simulink model "Sim_PMSM"  (R2023a)
settings: Solver=ode45  StartTime=0  StopTime=Stop_Time  MaxStep=Ts  RelTol=1e-3  EnableMultiTasking=on
values from neighbouring files (symbols this model uses):
  Bm = .018    (= 0.018)    [A_PMSM.m]
  Jm = 0.01    [A_PMSM.m]
  Lamf = 0.254    [A_PMSM.m]
  Lamf_Hat = 1.0*Lamf    (= 0.254)    [A_PMSM.m]
  Lds = 3.6e-3    (= 0.0036)    [A_PMSM.m]
  Lds_Hat = 1.0*Lds    (= 0.0036)    [A_PMSM.m]
  Lqs = 4.3e-3    (= 0.0043)    [A_PMSM.m]
  Lqs_Hat = 1.0*Lqs    (= 0.0043)    [A_PMSM.m]
  p = 3    [A_PMSM.m]
  Rs = 0.15    [A_PMSM.m]
  Step_Time = [0.1 0.2 0.3 0.4]    [A_PMSM.m]
  Stop_Time = 0.5    [A_PMSM.m]
  Te_Rated = interp1(MTPA.Is(Ind_PosTe),MTPA.Te(Ind_PosTe),Is_Rated)    [A_PMSM.m]
  Te_Ref_Set = ones(1,5)*Te_Rated    [A_PMSM.m]
  Te_SlewRate = inf    [A_PMSM.m]
  Thetarm_Init = 0*pi*1/p    (= 0)    [A_PMSM.m]
  TL = zeros(1,5)    [A_PMSM.m]
  Ts = 1/fs    (= 5e-05)    [A_PMSM.m]
  Tsw = 1/fsw    (= 0.0001)    [A_PMSM.m]
  Vdc = 310    [A_PMSM.m]
  Wrm_Fin = 10000*2*pi/60    (= 1047.1975512)    [A_PMSM.m]
  Wrm_Init = Wrpm_Ref_Set(1)*2*pi/60    [A_PMSM.m]
  Wrpm_Ref_Set = Wrm_Init*ones(1,5)    [A_PMSM.m]
undefined symbols (not defined in the file or in its folder): CC, DiscIntNeverNeededParam, FW, Mode, MTPA, SC
libraries: simulink x6
settings Model: SimulationMode=accelerator  Creator=KYC  LastModifiedBy=INHA
settings SolverCC: AlgebraicLoopSolver=TrustRegion
settings DataIOCC: LimitDataPoints=on  SaveFormat=Array  ReturnWorkspaceOutputs=off
settings OptimizationCC: LifeSpan=inf
settings DebuggingCC: UnderspecifiedInitializationDetection=Classic  MergeDetectMultiDrivingBlocksExec=none  SolverPrmCheckMsg=warning  InheritedTsInSrcMsg=none  UnconnectedInputMsg=warning  UnconnectedOutputMsg=warning  UnconnectedLineMsg=warning  AllowSymbolicDim=off  StateNameClashWarn=warning  SFUnexpectedBacktrackingDiag=warning  SFNoUnconditionalDefaultTransitionDiag=warning  SFExecutionAtInitializationDiag=none  ArithmeticOperatorsInVariantConditions=warning
settings HardwareCC: ProdBitPerPointer=32  ProdBitPerSizeT=32  ProdBitPerPtrDiffT=32  ProdLargestAtomicFloat=None  ProdIntDivRoundTo=Undefined  ProdEndianess=Unspecified  ProdWordSize=32  ProdHWDeviceType=32-bit Generic
settings ModelReferenceCC: EnableRefExpFcnMdlSchedulingChecks=on  PropagateSignalLabelsOutOfModel=off
settings SFSimCC: SimUseLocalCustomCode=off  CustomCodeUndefinedFunction=UseInterfaceOnly
settings RTWCC: RTWUseLocalCustomCode=off
settings CodeAppCC: StateflowObjectComments=on
settings GRTTargetCC: TargetLangStandard=C89/C90 (ANSI)
settings ConfigComp: CovMetricSettings=dw  CovSaveCumulativeToWorkspaceVar=on  CovSaveSingleToWorkspaceVar=on  CovExternalEMLEnable=off  CovSFcnEnable=off
settings SimscapeCC: SimscapeNormalizeSystem=off

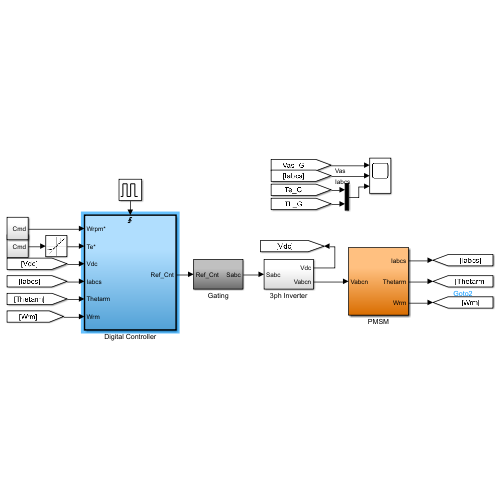
[thumbnail: Simulink's stored preview of the top-level diagram]
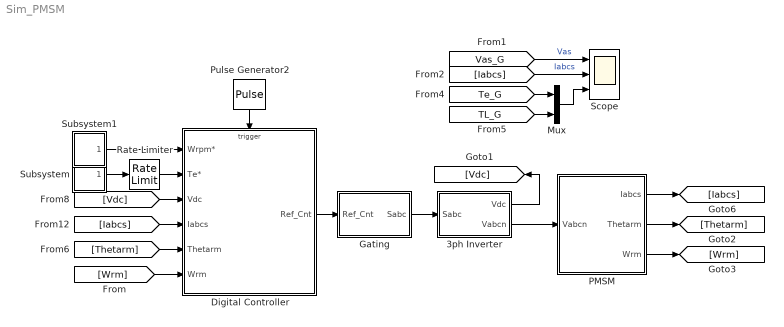
== system Sim_PMSM ==
  3ph Inverter : Subsystem
  Digital Controller : Subsystem
  Gating : Subsystem
  Mux : Mux  Inputs=2
  PMSM : Subsystem
  Pulse Generator2 : DiscretePulseGenerator  PulseType=Time based  Period=Ts  PulseWidth=50
  Rate Limiter : RateLimiter  RisingSlewLimit=Te_SlewRate*Te_Rated  FallingSlewLimit=-Te_SlewRate*Te_Rated  SampleTimeMode=inherited
  Scope : Scope  NumInputPorts=3
  Subsystem : Subsystem
  Subsystem1 : Subsystem
  wires:
  Pulse Generator2/1 -> Digital Controller/Trigger
  [Vdc] -> Digital Controller/3(Vdc)
  Digital Controller/1(Ref_Cnt) -> Gating/1(Ref_Cnt)
  [Thetarm] -> Digital Controller/5(Thetarm)
  PMSM/1(Iabcs) -> [Iabcs]
  Gating/1(Sabc) -> 3ph Inverter/1(Sabc)
  [Iabcs] -> Digital Controller/4(Iabcs)
  3ph Inverter/2(Vabcn) -> PMSM/1(Vabcn)
  3ph Inverter/1(Vdc) -> [Vdc]
  PMSM/2(Thetarm) -> [Thetarm]
  Subsystem/1(Cmd) -> Rate Limiter/1
  Subsystem1/1(Cmd) -> Digital Controller/1(Wrpm*)
  Rate Limiter/1 -> Digital Controller/2(Te*)
  PMSM/3(Wrm) -> [Wrm]
  [Wrm] -> Digital Controller/6(Wrm)
  [Te_G] -> Mux/1
  [TL_G] -> Mux/2
  [Vas_G] -> Scope/1  "Vas"
  [Iabcs] -> Scope/2  "Iabcs"
  Mux/1 -> Scope/3

== system Sim_PMSM/3ph Inverter ==
  Sabc : Inport
  Constant2 : Constant  Value=Vdc
  Gain : Gain  Gain=[1 0 0]  Multiplication=Matrix(K*u)
  Product1 : Product  RndMeth=Zero
  Relay2 : Relay  OnSwitchValue=0.5  OffSwitchValue=0.5  OnOutputValue=1/2  OffOutputValue=-1/2  OutDataTypeStr=double
  abcn to abcs : Subsystem
  Vdc : Outport
  Vabcn : Outport  Port=2
  tag scope: Vas_G=global
  wires:
  Constant2/1 -> Vdc/1, Product1/1
  Sabc/1 -> Relay2/1
  Relay2/1 -> Product1/2
  Product1/1 -> abcn to abcs/1(fabcn), Vabcn/1
  Gain/1 -> [Vas_G]
  abcn to abcs/1(fabcs) -> Gain/1

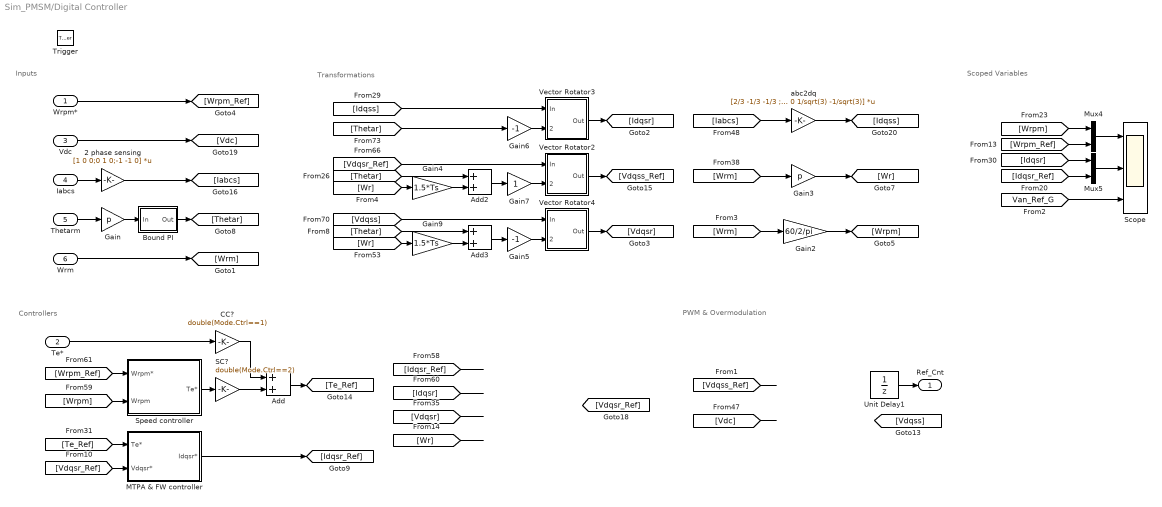
== system Sim_PMSM/Digital Controller ==
  note: PWM & Overmodulation
  note: Controllers
  note: Inputs
  note: Transformations
  note: Scoped Variables
  Wrpm* : Inport
  Te* : Inport  Port=2
  Vdc : Inport  Port=3
  Iabcs : Inport  Port=4
  Thetarm : Inport  Port=5
  Wrm : Inport  Port=6
  Trigger : TriggerPort  VariantControl=Variant
  2 phase sensing : Gain  Gain=[1 0 0;0 1 0;-1 -1 0]  Multiplication=Matrix(K*u)  SaturateOnIntegerOverflow=on  OutDataTypeStr=Inherit: Same as input  ParamDataTypeStr=Inherit: Same as input
  Add : Sum
  Add2 : Sum
  Add3 : Sum
  Bound PI : Subsystem
  CC? : Gain  Gain=double(Mode.Ctrl==1)
  Gain : Gain  Gain=p
  Gain2 : Gain  Gain=60/2/pi
  Gain3 : Gain  Gain=p
  Gain4 : Gain  Gain=1.5*Ts
  Gain5 : Gain  Gain=-1
  Gain6 : Gain  Gain=-1
  Gain7 : Gain
  Gain9 : Gain  Gain=1.5*Ts
  MTPA & FW controller : Subsystem
  Mux4 : Mux  Inputs=2
  Mux5 : Mux  Inputs=2
  SC? : Gain  Gain=double(Mode.Ctrl==2)
  Scope : Scope  NumInputPorts=3
  Speed controller : Subsystem
  Unit Delay1 : UnitDelay  SampleTime=-1  HasFrameUpgradeWarning=on
  Vector Rotator2 : Subsystem
  Vector Rotator3 : Subsystem
  Vector Rotator4 : Subsystem
  abc2dq : Gain  Gain=[2/3 -1/3 -1/3 ; 0 1/sqrt(3) -1/sqrt(3)]  Multiplication=Matrix(K*u)  SaturateOnIntegerOverflow=on  OutDataTypeStr=Inherit: Same as input  ParamDataTypeStr=Inherit: Same as input
  Ref_Cnt : Outport  InitialOutput=[0]
  wires:
  [Idqsr] -> ?
  abc2dq/1 -> [Idqss]
  [Iabcs] -> abc2dq/1
  Vdc/1 -> [Vdc]
  [Vdqsr] -> ?
  Gain3/1 -> [Wr]
  [Wrm] -> Gain3/1
  Wrpm*/1 -> [Wrpm_Ref]
  [Idqsr_Ref] -> ?
  [Wrpm_Ref] -> Speed controller/1(Wrpm*)
  [Wrpm] -> Speed controller/2(Wrpm)
  Thetarm/1 -> Gain/1
  [Wr] -> ?
  Gain/1 -> Bound PI/1(In)
  Bound PI/1(Out) -> [Thetar]
  ? -> [Vdqsr_Ref]
  Unit Delay1/1 -> Ref_Cnt/1
  ? -> [Vdqss]
  [Vdc] -> ?
  [Vdqsr_Ref] -> MTPA & FW controller/2(Vdqsr*)
  [Te_Ref] -> MTPA & FW controller/1(Te*)
  CC?/1 -> Add/1
  Speed controller/1(Te*) -> SC?/1
  Add/1 -> [Te_Ref]
  Add2/1 -> Gain7/1
  Gain7/1 -> Vector Rotator2/2(Theta)
  [Vdqsr_Ref] -> Vector Rotator2/1(In)
  Vector Rotator2/1(Out) -> [Vdqss_Ref]
  [Wr] -> Gain9/1
  Gain9/1 -> Add3/2
  Add3/1 -> Gain5/1
  [Thetar] -> Add3/1
  Gain5/1 -> Vector Rotator4/2(Theta)
  [Vdqss] -> Vector Rotator4/1(In)
  Vector Rotator4/1(Out) -> [Vdqsr]
  [Vdqss_Ref] -> ?
  Gain6/1 -> Vector Rotator3/2(Theta)
  [Idqss] -> Vector Rotator3/1(In)
  Vector Rotator3/1(Out) -> [Idqsr]
  [Thetar] -> Gain6/1
  ? -> Unit Delay1/1
  Iabcs/1 -> 2 phase sensing/1
  2 phase sensing/1 -> [Iabcs]
  MTPA & FW controller/1(Idqsr*) -> [Idqsr_Ref]
  [Wr] -> Gain4/1
  Gain4/1 -> Add2/2
  [Thetar] -> Add2/1
  [Idqsr] -> Mux5/1
  [Idqsr_Ref] -> Mux5/2
  [Wrpm] -> Mux4/1
  [Wrpm_Ref] -> Mux4/2
  SC?/1 -> Add/2
  Te*/1 -> CC?/1
  Wrm/1 -> [Wrm]
  [Wrm] -> Gain2/1
  Gain2/1 -> [Wrpm]
  Mux5/1 -> Scope/2
  [Van_Ref_G] -> Scope/3
  Mux4/1 -> Scope/1

== system Sim_PMSM/Gating ==
  Ref_Cnt : Inport
  Add3 : Sum  Inputs=+-
  Relay3 : Relay  OnSwitchValue=10*eps  OffSwitchValue=-10*eps  OutDataTypeStr=double
  Repeating Sequence1 : simulink/Sources/Repeating Sequence  rep_seq_t=[0 Tsw/2 Tsw]  rep_seq_y=[0 1 0]
  Sabc : Outport
  wires:
  Add3/1 -> Relay3/1
  Relay3/1 -> Sabc/1
  Repeating Sequence1/1 -> Add3/2
  Ref_Cnt/1 -> Add3/1

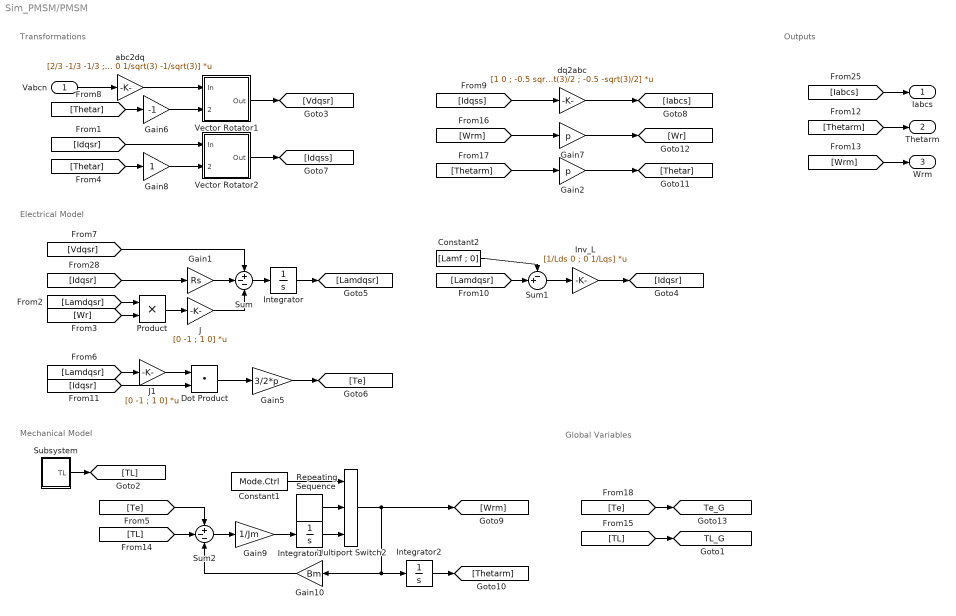
== system Sim_PMSM/PMSM ==
  note: Transformations
  note: Electrical Model
  note: Mechanical Model
  note: Global Variables
  note: Outputs
  Vabcn : Inport
  Constant1 : Constant  Value=Mode.Ctrl
  Constant2 : Constant  Value=[Lamf ; 0]
  Dot Product : DotProduct  OutDataTypeStr=Inherit: Inherit via internal rule
  Gain1 : Gain  Gain=Rs
  Gain10 : Gain  Gain=Bm
  Gain2 : Gain  Gain=p
  Gain5 : Gain  Gain=3/2*p
  Gain6 : Gain  Gain=-1
  Gain7 : Gain  Gain=p
  Gain8 : Gain
  Gain9 : Gain  Gain=1/Jm
  Integrator : Integrator  InitialCondition=[Lamf ; 0]
  Integrator1 : Integrator  InitialCondition=Wrm_Init
  Integrator2 : Integrator  InitialCondition=Thetarm_Init  WrapState=on
  Inv_L : Gain  Gain=[1/Lds 0 ; 0 1/Lqs]  Multiplication=Matrix(K*u)
  J : Gain  Gain=[0 -1 ; 1 0]  Multiplication=Matrix(K*u)
  J1 : Gain  Gain=[0 -1 ; 1 0]  Multiplication=Matrix(K*u)
  Multiport Switch2 : MultiPortSwitch  Inputs=2  OutDataTypeStr=double  SaturateOnIntegerOverflow=off  InputSameDT=off
  Product : Product  RndMeth=Zero
  Repeating Sequence : simulink/Sources/Repeating Sequence  rep_seq_t=[0 Stop_Time]  rep_seq_y=[Wrm_Init Wrm_Fin]
  Subsystem : Subsystem
  Sum : Sum  Inputs=+--
  Sum1 : Sum  Inputs=-+|
  Sum2 : Sum  Inputs=+--
  Vector Rotator1 : Subsystem
  Vector Rotator2 : Subsystem
  abc2dq : Gain  Gain=[2/3 -1/3 -1/3 ; 0 1/sqrt(3) -1/sqrt(3)]  Multiplication=Matrix(K*u)  SaturateOnIntegerOverflow=on  OutDataTypeStr=Inherit: Same as input  ParamDataTypeStr=Inherit: Same as input
  dq2abc : Gain  Gain=[1 0 ; -0.5 sqrt(3)/2 ; -0.5 -sqrt(3)/2]  Multiplication=Matrix(K*u)
  Iabcs : Outport
  Thetarm : Outport  Port=2
  Wrm : Outport  Port=3
  tag scope: TL_G=global, Te_G=global
  wires:
  [Iabcs] -> Iabcs/1
  [Wrm] -> Gain7/1
  [Thetarm] -> Gain2/1
  Gain7/1 -> [Wr]
  dq2abc/1 -> [Iabcs]
  [Idqss] -> dq2abc/1
  Vector Rotator2/1(Out) -> [Idqss]
  Vabcn/1 -> abc2dq/1
  abc2dq/1 -> Vector Rotator1/1(In)
  [Idqsr] -> Vector Rotator2/1(In)
  Vector Rotator1/1(Out) -> [Vdqsr]
  [Thetarm] -> Thetarm/1
  Gain2/1 -> [Thetar]
  [Thetar] -> Gain6/1
  Gain6/1 -> Vector Rotator1/2(Theta)
  [Thetar] -> Gain8/1
  Gain8/1 -> Vector Rotator2/2(Theta)
  Gain10/1 -> Sum2/3
  Integrator2/1 -> [Thetarm]
  [Te] -> Sum2/1
  Sum2/1 -> Gain9/1
  Multiport Switch2/1 -> [Wrm], Integrator2/1, Gain10/1
  Gain9/1 -> Integrator1/1
  Constant1/1 -> Multiport Switch2/1
  Sum1/1 -> Inv_L/1
  Inv_L/1 -> [Idqsr]
  [Lamdqsr] -> Sum1/2
  Constant2/1 -> Sum1/1
  Dot Product/1 -> Gain5/1
  J1/1 -> Dot Product/1
  [Lamdqsr] -> J1/1
  [Idqsr] -> Dot Product/2
  Gain5/1 -> [Te]
  Integrator/1 -> [Lamdqsr]
  [Vdqsr] -> Sum/1
  [Lamdqsr] -> Product/1
  Sum/1 -> Integrator/1
  [Wr] -> Product/2
  Product/1 -> J/1
  [Idqsr] -> Gain1/1
  J/1 -> Sum/3
  Gain1/1 -> Sum/2
  Integrator1/1 -> Multiport Switch2/3
  Repeating Sequence/1 -> Multiport Switch2/2
  [Wrm] -> Wrm/1
  Subsystem/1(TL) -> [TL]
  [TL] -> Sum2/2
  [TL] -> [TL_G]
  [Te] -> [Te_G]

== system Sim_PMSM/Subsystem ==
  Add : Sum  Inputs=++++
  Step1 : Step  Time=Step_Time(1)  Before=Te_Ref_Set(1)  After=Te_Ref_Set(2)
  Step2 : Step  Time=Step_Time(3)  After=Te_Ref_Set(4)-Te_Ref_Set(3)
  Step3 : Step  Time=Step_Time(2)  After=Te_Ref_Set(3)-Te_Ref_Set(2)
  Step4 : Step  Time=Step_Time(4)  After=Te_Ref_Set(5)-Te_Ref_Set(4)
  Cmd : Outport
  wires:
  Add/1 -> Cmd/1
  Step2/1 -> Add/3
  Step4/1 -> Add/4
  Step3/1 -> Add/2
  Step1/1 -> Add/1

== system Sim_PMSM/Subsystem1 ==
  Add : Sum  Inputs=++++
  Step1 : Step  Time=Step_Time(1)  Before=Wrpm_Ref_Set(1)  After=Wrpm_Ref_Set(2)
  Step2 : Step  Time=Step_Time(3)  After=Wrpm_Ref_Set(4)-Wrpm_Ref_Set(3)
  Step3 : Step  Time=Step_Time(2)  After=Wrpm_Ref_Set(3)-Wrpm_Ref_Set(2)
  Step4 : Step  Time=Step_Time(4)  After=Wrpm_Ref_Set(5)-Wrpm_Ref_Set(4)
  Cmd : Outport
  wires:
  Step1/1 -> Add/1
  Step3/1 -> Add/2
  Step4/1 -> Add/4
  Step2/1 -> Add/3
  Add/1 -> Cmd/1

== system Sim_PMSM/3ph Inverter/abcn to abcs ==
  fabcn : Inport
  Add1 : Sum  Inputs=+-
  Gain2 : Gain  Gain=1/3
  Sum of Elements : Sum  Inputs=+
  fabcs : Outport
  wires:
  Gain2/1 -> Add1/2
  Add1/1 -> fabcs/1
  Sum of Elements/1 -> Gain2/1
  fabcn/1 -> Add1/1, Sum of Elements/1

== system Sim_PMSM/Digital Controller/Bound PI ==
  In : Inport
  Fcn1 : Fcn  Expr=1/(2*pi)*u+0.5
  Fcn2 : Fcn  Expr=u-floor(u)
  Fcn3 : Fcn  Expr=2*pi*(u-0.5)
  Out : Outport
  wires:
  Fcn1/1 -> Fcn2/1
  Fcn2/1 -> Fcn3/1
  In/1 -> Fcn1/1
  Fcn3/1 -> Out/1

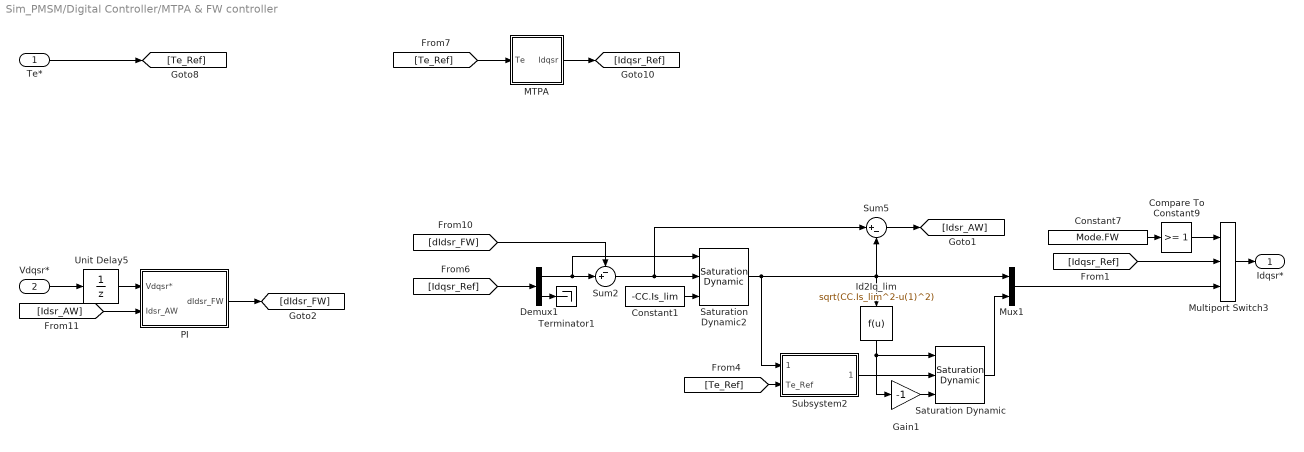
== system Sim_PMSM/Digital Controller/MTPA & FW controller ==
  Te* : Inport
  Vdqsr* : Inport  Port=2
  Compare To Constant9 : simulink/Logic and Bit Operations/Compare To Constant  relop=>=  const=1  OutDataTypeStr=boolean
  Constant1 : Constant  Value=-CC.Is_lim
  Constant7 : Constant  Value=Mode.FW
  Demux1 : Demux  Outputs=2
  Gain1 : Gain  Gain=-1
  Id2Iq_lim : Fcn  Expr=sqrt(CC.Is_lim^2-u(1)^2)
  MTPA : Subsystem
  Multiport Switch3 : MultiPortSwitch  DataPortOrder=Zero-based contiguous  Inputs=2  zeroidx=on  OutDataTypeStr=double  SaturateOnIntegerOverflow=off  InputSameDT=off
  Mux1 : Mux  Inputs=[1 1]
  PI : Subsystem
  Saturation Dynamic : simulink/Discontinuities/Saturation Dynamic  OutMin=[]  OutMax=[]  OutDataTypeStr=Inherit: Same as second input  OutDataType=fixdt(1, 16)  OutScaling=2^-10  DoSatur=off
  Saturation Dynamic2 : simulink/Discontinuities/Saturation Dynamic  OutMin=[]  OutMax=[]  OutDataTypeStr=Inherit: Same as second input  OutDataType=fixdt(1, 16)  OutScaling=2^-10  DoSatur=off
  Subsystem2 : Subsystem
  Sum2 : Sum  Inputs=-+|
  Sum5 : Sum  Inputs=|+-
  Terminator1 : Terminator
  Unit Delay5 : UnitDelay  SampleTime=-1  HasFrameUpgradeWarning=on
  Idqsr* : Outport
  wires:
  Demux1/1 -> Saturation Dynamic2/1, Sum2/2
  Saturation Dynamic2/1 -> Subsystem2/1(Idsr_Ref), Sum5/2, Id2Iq_lim/1, Mux1/1
  Saturation Dynamic/1 -> Mux1/2
  Id2Iq_lim/1 -> Saturation Dynamic/1, Gain1/1
  Gain1/1 -> Saturation Dynamic/3
  Sum2/1 -> Saturation Dynamic2/2, Sum5/1
  [Idqsr_Ref] -> Demux1/1
  Te*/1 -> [Te_Ref]
  [Te_Ref] -> MTPA/1(Te)
  MTPA/1(Idqsr) -> [Idqsr_Ref]
  Vdqsr*/1 -> Unit Delay5/1
  [Te_Ref] -> Subsystem2/2(Te_Ref)
  Constant1/1 -> Saturation Dynamic2/3
  [dIdsr_FW] -> Sum2/1
  Sum5/1 -> [Idsr_AW]
  [Idsr_AW] -> PI/2(Idsr_AW)
  Unit Delay5/1 -> PI/1(Vdqsr*)
  Subsystem2/1(Iqsr_Ref) -> Saturation Dynamic/2
  Constant7/1 -> Compare To Constant9/1
  Compare To Constant9/1 -> Multiport Switch3/1
  Multiport Switch3/1 -> Idqsr*/1
  [Idqsr_Ref] -> Multiport Switch3/2
  Mux1/1 -> Multiport Switch3/3
  Demux1/2 -> Terminator1/1
  PI/1(dIdsr_FW) -> [dIdsr_FW]

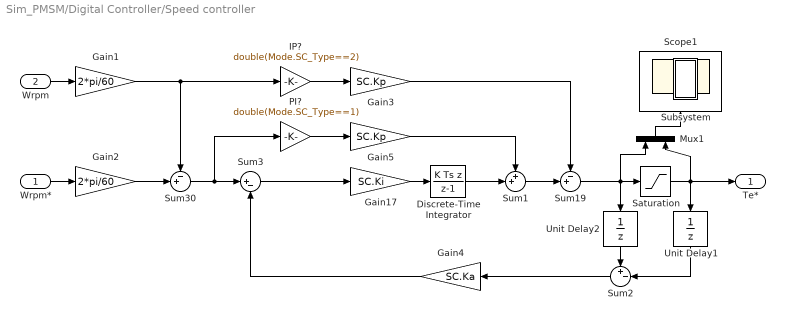
== system Sim_PMSM/Digital Controller/Speed controller ==
  Wrpm* : Inport
  Wrpm : Inport  Port=2
  Discrete-Time Integrator : DiscreteIntegrator  IntegratorMethod=Integration: Backward Euler  InitialCondition=double(Mode.SC_Type==2)*SC.Kp*Wrm_Init+TL(1)  SampleTime=-1  ICPrevOutput=DiscIntNeverNeededParam  ICPrevScaledInput=DiscIntNeverNeededParam
  Gain1 : Gain  Gain=2*pi/60
  Gain17 : Gain  Gain=SC.Ki
  Gain2 : Gain  Gain=2*pi/60
  Gain3 : Gain  Gain=SC.Kp
  Gain4 : Gain  Gain=SC.Ka
  Gain5 : Gain  Gain=SC.Kp
  IP? : Gain  Gain=double(Mode.SC_Type==2)
  Mux1 : Mux  Inputs=2
  PI? : Gain  Gain=double(Mode.SC_Type==1)
  Saturation : Saturate  UpperLimit=SC.Te_lim  LowerLimit=-SC.Te_lim
  Scope1 : Scope
  Subsystem : Subsystem
  Sum1 : Sum  Inputs=++|
  Sum19 : Sum  Inputs=-+|
  Sum2 : Sum  Inputs=+-|
  Sum3 : Sum  Inputs=|+-
  Sum30 : Sum  Inputs=-+|
  Unit Delay1 : UnitDelay  SampleTime=-1  HasFrameUpgradeWarning=on
  Unit Delay2 : UnitDelay  SampleTime=-1  HasFrameUpgradeWarning=on
  Te* : Outport  InitialOutput=[0]
  wires:
  Gain2/1 -> Sum30/2
  Mux1/1 -> Scope1/1
  Gain17/1 -> Discrete-Time Integrator/1
  Gain3/1 -> Sum19/1
  Sum3/1 -> Gain17/1
  Sum30/1 -> PI?/1, Sum3/1
  Unit Delay2/1 -> Sum2/1
  Gain4/1 -> Sum3/2
  Saturation/1 -> Te*/1, Mux1/2, Unit Delay1/1
  Sum19/1 -> Saturation/1, Mux1/1, Unit Delay2/1
  Sum2/1 -> Gain4/1
  Unit Delay1/1 -> Sum2/2
  Gain1/1 -> Sum30/1, IP?/1
  Wrpm*/1 -> Gain2/1
  Wrpm/1 -> Gain1/1
  Discrete-Time Integrator/1 -> Sum1/2
  Sum1/1 -> Sum19/2
  Gain5/1 -> Sum1/1
  IP?/1 -> Gain3/1
  PI?/1 -> Gain5/1

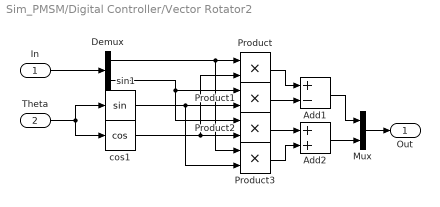
== system Sim_PMSM/Digital Controller/Vector Rotator2 ==
  In : Inport
  Theta : Inport  Port=2
  Add1 : Sum  Inputs=+-
  Add2 : Sum
  Demux : Demux  Outputs=2
  Mux : Mux  Inputs=[1 1]
  Product{,1..3} (4 alike) : Product  RndMeth=Zero
  cos1 : Trigonometry  Operator=cos
  sin1 : Trigonometry
  Out : Outport
  wires:
  Theta/1 -> cos1/1, sin1/1
  Demux/1 -> Product3/1, Product/1
  Mux/1 -> Out/1
  In/1 -> Demux/1
  Demux/2 -> Product1/1, Product2/1
  cos1/1 -> Product/2, Product2/2
  sin1/1 -> Product1/2, Product3/2
  Product/1 -> Add1/1
  Product1/1 -> Add1/2
  Add1/1 -> Mux/1
  Product2/1 -> Add2/1
  Product3/1 -> Add2/2
  Add2/1 -> Mux/2

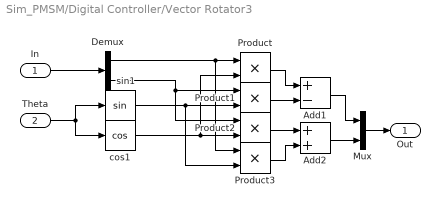
== system Sim_PMSM/Digital Controller/Vector Rotator3 ==
  In : Inport
  Theta : Inport  Port=2
  Add1 : Sum  Inputs=+-
  Add2 : Sum
  Demux : Demux  Outputs=2
  Mux : Mux  Inputs=[1 1]
  Product{,1..3} (4 alike) : Product  RndMeth=Zero
  cos1 : Trigonometry  Operator=cos
  sin1 : Trigonometry
  Out : Outport
  wires:
  Theta/1 -> cos1/1, sin1/1
  Demux/1 -> Product3/1, Product/1
  Mux/1 -> Out/1
  In/1 -> Demux/1
  Demux/2 -> Product1/1, Product2/1
  cos1/1 -> Product/2, Product2/2
  sin1/1 -> Product1/2, Product3/2
  Product/1 -> Add1/1
  Product1/1 -> Add1/2
  Add1/1 -> Mux/1
  Product2/1 -> Add2/1
  Product3/1 -> Add2/2
  Add2/1 -> Mux/2

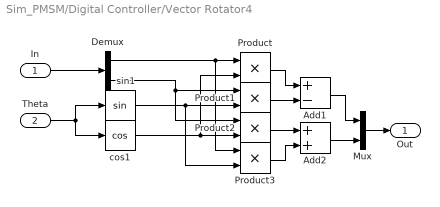
== system Sim_PMSM/Digital Controller/Vector Rotator4 ==
  In : Inport
  Theta : Inport  Port=2
  Add1 : Sum  Inputs=+-
  Add2 : Sum
  Demux : Demux  Outputs=2
  Mux : Mux  Inputs=[1 1]
  Product{,1..3} (4 alike) : Product  RndMeth=Zero
  cos1 : Trigonometry  Operator=cos
  sin1 : Trigonometry
  Out : Outport
  wires:
  Add2/1 -> Mux/2
  Product3/1 -> Add2/2
  Product2/1 -> Add2/1
  Add1/1 -> Mux/1
  Product1/1 -> Add1/2
  Product/1 -> Add1/1
  sin1/1 -> Product3/2, Product1/2
  cos1/1 -> Product2/2, Product/2
  Demux/2 -> Product2/1, Product1/1
  In/1 -> Demux/1
  Mux/1 -> Out/1
  Demux/1 -> Product/1, Product3/1
  Theta/1 -> sin1/1, cos1/1

== system Sim_PMSM/PMSM/Subsystem ==
  Add : Sum  Inputs=++++
  Step1 : Step  Time=Step_Time(1)  Before=TL(1)  After=TL(2)
  Step2 : Step  Time=Step_Time(3)  After=TL(4)-TL(3)
  Step3 : Step  Time=Step_Time(2)  After=TL(3)-TL(2)
  Step4 : Step  Time=Step_Time(4)  After=TL(5)-TL(4)
  TL : Outport
  wires:
  Add/1 -> TL/1
  Step2/1 -> Add/3
  Step4/1 -> Add/4
  Step3/1 -> Add/2
  Step1/1 -> Add/1

== system Sim_PMSM/PMSM/Vector Rotator1 ==
  In : Inport
  Theta : Inport  Port=2
  Add1 : Sum  Inputs=+-
  Add2 : Sum
  Demux : Demux  Outputs=2
  Mux : Mux  Inputs=[1 1]
  Product{,1..3} (4 alike) : Product  RndMeth=Zero
  cos1 : Trigonometry  Operator=cos
  sin1 : Trigonometry
  Out : Outport
  wires:
  Add2/1 -> Mux/2
  Product3/1 -> Add2/2
  Product2/1 -> Add2/1
  Add1/1 -> Mux/1
  Product1/1 -> Add1/2
  Product/1 -> Add1/1
  sin1/1 -> Product3/2, Product1/2
  cos1/1 -> Product2/2, Product/2
  Demux/2 -> Product2/1, Product1/1
  In/1 -> Demux/1
  Mux/1 -> Out/1
  Demux/1 -> Product/1, Product3/1
  Theta/1 -> sin1/1, cos1/1

== system Sim_PMSM/PMSM/Vector Rotator2 ==
  In : Inport
  Theta : Inport  Port=2
  Add1 : Sum  Inputs=+-
  Add2 : Sum
  Demux : Demux  Outputs=2
  Mux : Mux  Inputs=[1 1]
  Product{,1..3} (4 alike) : Product  RndMeth=Zero
  cos1 : Trigonometry  Operator=cos
  sin1 : Trigonometry
  Out : Outport
  wires:
  Theta/1 -> cos1/1, sin1/1
  Demux/1 -> Product3/1, Product/1
  Mux/1 -> Out/1
  In/1 -> Demux/1
  Demux/2 -> Product1/1, Product2/1
  cos1/1 -> Product/2, Product2/2
  sin1/1 -> Product1/2, Product3/2
  Product/1 -> Add1/1
  Product1/1 -> Add1/2
  Add1/1 -> Mux/1
  Product2/1 -> Add2/1
  Product3/1 -> Add2/2
  Add2/1 -> Mux/2

== system Sim_PMSM/Digital Controller/MTPA & FW controller/MTPA ==
  Te : Inport
  1-D Lookup Table : Lookup_n-D  NumberOfTableDimensions=1  BreakpointsForDimension1=MTPA.Te  Table=MTPA.Iqsr  InternalRulePriority=Speed  RndMeth=Simplest
  1-D Lookup Table1 : Lookup_n-D  NumberOfTableDimensions=1  BreakpointsForDimension1=MTPA.Te  Table=MTPA.Idsr  InternalRulePriority=Speed  RndMeth=Simplest
  Mux : Mux  Inputs=2
  Idqsr : Outport
  wires:
  Te/1 -> 1-D Lookup Table1/1, 1-D Lookup Table/1
  Mux/1 -> Idqsr/1
  1-D Lookup Table1/1 -> Mux/1
  1-D Lookup Table/1 -> Mux/2

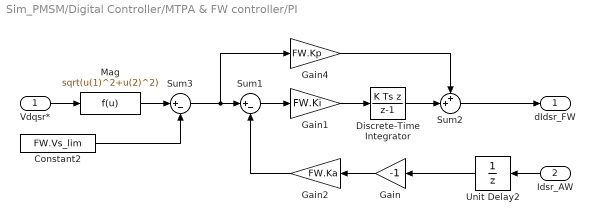
== system Sim_PMSM/Digital Controller/MTPA & FW controller/PI ==
  Vdqsr* : Inport
  Idsr_AW : Inport  Port=2
  Constant2 : Constant  Value=FW.Vs_lim
  Discrete-Time Integrator : DiscreteIntegrator  IntegratorMethod=Integration: Backward Euler  SampleTime=-1  ICPrevOutput=DiscIntNeverNeededParam  ICPrevScaledInput=DiscIntNeverNeededParam
  Gain : Gain  Gain=-1
  Gain1 : Gain  Gain=FW.Ki
  Gain2 : Gain  Gain=FW.Ka
  Gain4 : Gain  Gain=FW.Kp
  Mag : Fcn  Expr=sqrt(u(1)^2+u(2)^2)
  Sum1 : Sum  Inputs=|+-
  Sum2 : Sum  Inputs=++|
  Sum3 : Sum  Inputs=|+-
  Unit Delay2 : UnitDelay  SampleTime=-1  HasFrameUpgradeWarning=on
  dIdsr_FW : Outport
  wires:
  Gain/1 -> Gain2/1
  Idsr_AW/1 -> Unit Delay2/1
  Sum3/1 -> Gain4/1, Sum1/1
  Gain1/1 -> Discrete-Time Integrator/1
  Sum1/1 -> Gain1/1
  Discrete-Time Integrator/1 -> Sum2/2
  Gain4/1 -> Sum2/1
  Sum2/1 -> dIdsr_FW/1
  Mag/1 -> Sum3/1
  Constant2/1 -> Sum3/2
  Vdqsr*/1 -> Mag/1
  Unit Delay2/1 -> Gain/1
  Gain2/1 -> Sum1/2

== system Sim_PMSM/Digital Controller/MTPA & FW controller/Subsystem2 ==
  Idsr_Ref : Inport
  Te_Ref : Inport  Port=2
  Add1 : Sum
  Constant : Constant  Value=Lamf_Hat
  Divide : Product  Inputs=*/
  Gain2 : Gain  Gain=2/3/p
  Gain5 : Gain  Gain=Lds_Hat-Lqs_Hat
  Iqsr_Ref : Outport
  wires:
  Gain5/1 -> Add1/1
  Te_Ref/1 -> Gain2/1
  Constant/1 -> Add1/2
  Gain2/1 -> Divide/1
  Add1/1 -> Divide/2
  Idsr_Ref/1 -> Gain5/1
  Divide/1 -> Iqsr_Ref/1

== system Sim_PMSM/Digital Controller/Speed controller/Subsystem ==
  Current controller : Subsystem
  PWM : Subsystem

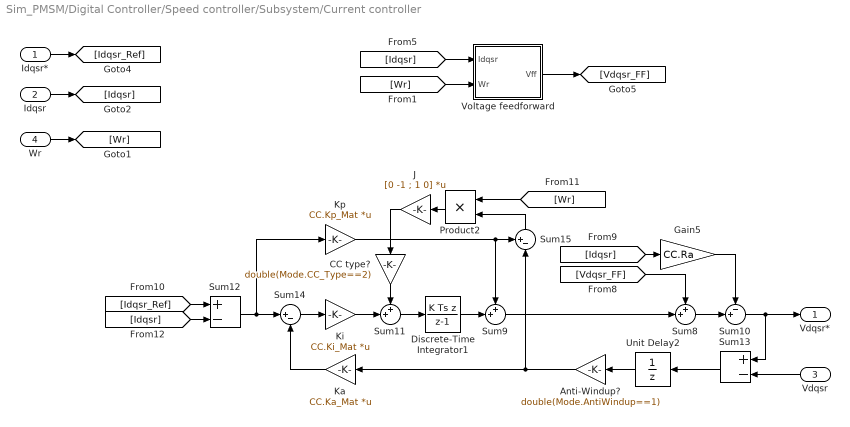
== system Sim_PMSM/Digital Controller/Speed controller/Subsystem/Current controller ==
  Idqsr* : Inport
  Idqsr : Inport  Port=2
  Vdqsr : Inport  Port=3
  Wr : Inport  Port=4
  Anti-Windup? : Gain  Gain=double(Mode.AntiWindup==1)
  CC type? : Gain  Gain=double(Mode.CC_Type==2)
  Discrete-Time Integrator1 : DiscreteIntegrator  IntegratorMethod=Integration: Backward Euler  SampleTime=-1  ICPrevOutput=DiscIntNeverNeededParam  ICPrevScaledInput=DiscIntNeverNeededParam
  Gain5 : Gain  Gain=CC.Ra
  J : Gain  Gain=[0 -1 ; 1 0]  Multiplication=Matrix(K*u)
  Ka : Gain  Gain=CC.Ka_Mat  Multiplication=Matrix(K*u)  SaturateOnIntegerOverflow=on  OutDataTypeStr=Inherit: Same as input  ParamDataTypeStr=Inherit: Same as input
  Ki : Gain  Gain=CC.Ki_Mat  Multiplication=Matrix(K*u)  SaturateOnIntegerOverflow=on  OutDataTypeStr=Inherit: Same as input  ParamDataTypeStr=Inherit: Same as input
  Kp : Gain  Gain=CC.Kp_Mat  Multiplication=Matrix(K*u)  SaturateOnIntegerOverflow=on  OutDataTypeStr=Inherit: Same as input  ParamDataTypeStr=Inherit: Same as input
  Product2 : Product  RndMeth=Zero
  Sum10 : Sum  Inputs=-+|
  Sum11 : Sum  Inputs=++|
  Sum12 : Sum  Inputs=+-
  Sum13 : Sum  Inputs=+-
  Sum14 : Sum  Inputs=|+-
  Sum15 : Sum  Inputs=+-|
  Sum8 : Sum  Inputs=++|
  Sum9 : Sum  Inputs=++|
  Unit Delay2 : UnitDelay  SampleTime=-1  HasFrameUpgradeWarning=on
  Voltage feedforward : Subsystem
  Vdqsr* : Outport
  wires:
  Idqsr/1 -> [Idqsr]
  Idqsr*/1 -> [Idqsr_Ref]
  Wr/1 -> [Wr]
  [Idqsr] -> Voltage feedforward/1(Idqsr)
  [Wr] -> Voltage feedforward/2(Wr)
  Voltage feedforward/1(Vff) -> [Vdqsr_FF]
  Discrete-Time Integrator1/1 -> Sum9/2
  Gain5/1 -> Sum10/1
  [Idqsr_Ref] -> Sum12/1
  Sum11/1 -> Discrete-Time Integrator1/1
  Ki/1 -> Sum11/2
  Kp/1 -> Sum15/1, Sum9/1
  Sum8/1 -> Sum10/2
  CC type?/1 -> Sum11/1
  [Idqsr] -> Gain5/1
  J/1 -> CC type?/1
  Product2/1 -> J/1
  Sum12/1 -> Sum14/1, Kp/1
  [Idqsr] -> Sum12/2
  Sum9/1 -> Sum8/2
  [Wr] -> Product2/1
  [Vdqsr_FF] -> Sum8/1
  Sum10/1 -> Vdqsr*/1, Sum13/1
  Vdqsr/1 -> Sum13/2
  Unit Delay2/1 -> Anti-Windup?/1
  Sum13/1 -> Unit Delay2/1
  Sum14/1 -> Ki/1
  Ka/1 -> Sum14/2
  Anti-Windup?/1 -> Sum15/2, Ka/1
  Sum15/1 -> Product2/2

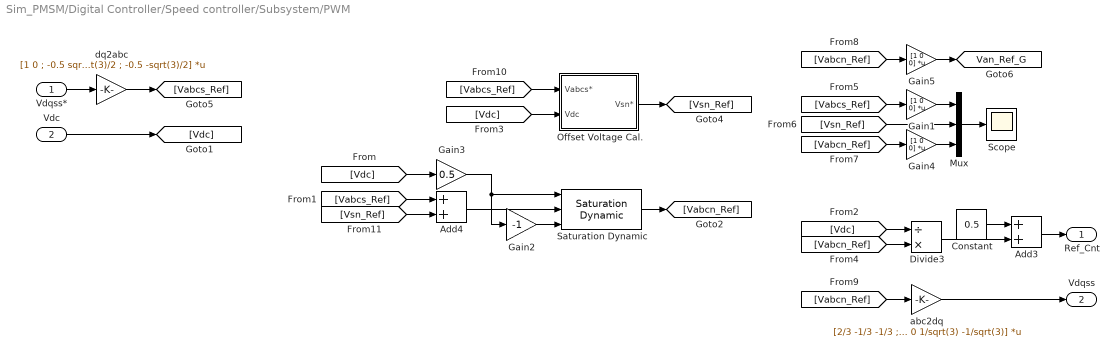
== system Sim_PMSM/Digital Controller/Speed controller/Subsystem/PWM ==
  Vdqss* : Inport
  Vdc : Inport  Port=2
  Add3 : Sum
  Add4 : Sum
  Constant : Constant  Value=0.5
  Divide3 : Product  Inputs=/*
  Gain1 : Gain  Gain=[1 0 0]  Multiplication=Matrix(K*u)
  Gain2 : Gain  Gain=-1
  Gain3 : Gain  Gain=0.5
  Gain4 : Gain  Gain=[1 0 0]  Multiplication=Matrix(K*u)
  Gain5 : Gain  Gain=[1 0 0]  Multiplication=Matrix(K*u)
  Mux : Mux  Inputs=3
  Offset Voltage Cal. : Subsystem
  Saturation Dynamic : simulink/Discontinuities/Saturation Dynamic  OutMin=[]  OutMax=[]  OutDataTypeStr=Inherit: Same as second input  OutDataType=fixdt(1, 16)  OutScaling=2^-10  DoSatur=off
  Scope : Scope
  abc2dq : Gain  Gain=[2/3 -1/3 -1/3 ; 0 1/sqrt(3) -1/sqrt(3)]  Multiplication=Matrix(K*u)  SaturateOnIntegerOverflow=on  OutDataTypeStr=Inherit: Same as input  ParamDataTypeStr=Inherit: Same as input
  dq2abc : Gain  Gain=[1 0 ; -0.5 sqrt(3)/2 ; -0.5 -sqrt(3)/2]  Multiplication=Matrix(K*u)
  Ref_Cnt : Outport
  Vdqss : Outport  Port=2
  tag scope: Van_Ref_G=global
  wires:
  Vdqss*/1 -> dq2abc/1
  dq2abc/1 -> [Vabcs_Ref]
  [Vabcs_Ref] -> Add4/1
  [Vsn_Ref] -> Add4/2
  Gain3/1 -> Saturation Dynamic/1, Gain2/1
  Gain2/1 -> Saturation Dynamic/3
  Add4/1 -> Saturation Dynamic/2
  Vdc/1 -> [Vdc]
  [Vdc] -> Gain3/1
  Mux/1 -> Scope/1
  [Vabcs_Ref] -> Gain1/1
  Gain1/1 -> Mux/1
  [Vsn_Ref] -> Mux/2
  Gain4/1 -> Mux/3
  [Vabcn_Ref] -> Gain4/1
  Saturation Dynamic/1 -> [Vabcn_Ref]
  abc2dq/1 -> Vdqss/1
  [Vabcn_Ref] -> abc2dq/1
  [Vabcs_Ref] -> Offset Voltage Cal./1(Vabcs*)
  [Vdc] -> Offset Voltage Cal./2(Vdc)
  Offset Voltage Cal./1(Vsn*) -> [Vsn_Ref]
  Divide3/1 -> Add3/2
  [Vabcn_Ref] -> Divide3/2
  Constant/1 -> Add3/1
  Add3/1 -> Ref_Cnt/1
  [Vdc] -> Divide3/1
  Gain5/1 -> [Van_Ref_G]
  [Vabcn_Ref] -> Gain5/1

== system Sim_PMSM/Digital Controller/Speed controller/Subsystem/Current controller/Voltage feedforward ==
  Idqsr : Inport
  Wr : Inport  Port=2
  CC type : Gain  Gain=double(Mode.CC_Type==1)
  Constant : Constant  Value=[Lamf_Hat;0]
  J : Gain  Gain=[0 -1 ; 1 0]  Multiplication=Matrix(K*u)
  L_Hat : Gain  Gain=[Lds_Hat 0 ; 0 Lqs_Hat]  Multiplication=Matrix(K*u)
  Product : Product  RndMeth=Zero
  Sum2 : Sum  Inputs=|++
  Vff : Outport
  wires:
  Idqsr/1 -> L_Hat/1
  Wr/1 -> Product/2
  J/1 -> Product/1
  Product/1 -> Vff/1
  L_Hat/1 -> CC type/1
  Sum2/1 -> J/1
  CC type/1 -> Sum2/1
  Constant/1 -> Sum2/2

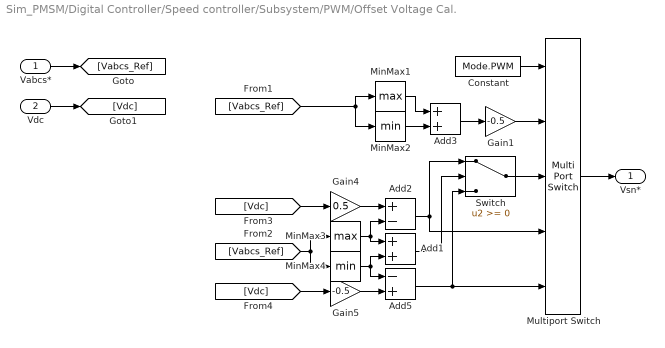
== system Sim_PMSM/Digital Controller/Speed controller/Subsystem/PWM/Offset Voltage Cal. ==
  Vabcs* : Inport
  Vdc : Inport  Port=2
  Add1 : Sum
  Add2 : Sum  Inputs=+-
  Add3 : Sum
  Add5 : Sum  Inputs=-+
  Constant : Constant  Value=Mode.PWM
  Gain1 : Gain  Gain=-0.5
  Gain4 : Gain  Gain=0.5
  Gain5 : Gain  Gain=-0.5
  MinMax1 : MinMax  Function=max
  MinMax2 : MinMax
  MinMax3 : MinMax  Function=max
  MinMax4 : MinMax
  Multiport Switch : MultiPortSwitch  Inputs=4  SaturateOnIntegerOverflow=off  InputSameDT=off
  Switch : Switch  SaturateOnIntegerOverflow=off  InputSameDT=off
  Vsn* : Outport
  wires:
  Add2/1 -> Multiport Switch/4, Switch/1
  Add3/1 -> Gain1/1
  MinMax2/1 -> Add3/2
  MinMax1/1 -> Add3/1
  Constant/1 -> Multiport Switch/1
  Gain1/1 -> Multiport Switch/2
  MinMax3/1 -> Add2/2, Add1/1
  [Vabcs_Ref] -> MinMax3/1, MinMax4/1
  [Vabcs_Ref] -> MinMax2/1, MinMax1/1
  Multiport Switch/1 -> Vsn*/1
  Add1/1 -> Switch/2
  MinMax4/1 -> Add1/2, Add5/1
  Gain4/1 -> Add2/1
  Switch/1 -> Multiport Switch/3
  [Vdc] -> Gain5/1
  Gain5/1 -> Add5/2
  Add5/1 -> Switch/3, Multiport Switch/5
  [Vdc] -> Gain4/1
  Vabcs*/1 -> [Vabcs_Ref]
  Vdc/1 -> [Vdc]
